simulink model "quadrotor"  (R2018b)
settings: Solver=ode4  StartTime=0.0  StopTime=inf  FixedStep=dt  RelTol=1e-3
values from neighbouring files (symbols this model uses):
  dt = 0.001    [InitSimulation.m]
  gravity = 9.81    [modelParameters.m]
  vehicle =     [Quadcopter-250mm-0.6kg-15min-EMAX.mat]    (also in Quadcopter-450mm-1.5kg-7min-DJI.mat)
libraries: simulink_extras x1

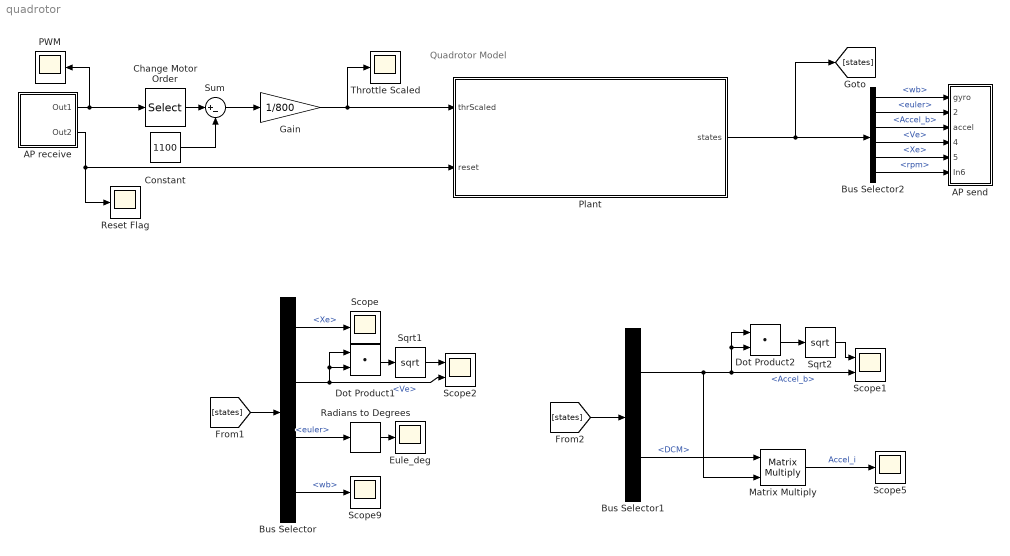
== system quadrotor ==
  note: Quadrotor Model
  AP receive : Subsystem  AncestorBlock=AP_Conector/AP receive
  AP send : Subsystem  AncestorBlock=AP_Conector/AP send
  Bus Selector : BusSelector  OutputSignals=Xe,Ve,euler,wb
  Bus Selector1 : BusSelector  OutputSignals=Accel_b,DCM
  Bus Selector2 : BusSelector  OutputSignals=wb,euler,Accel_b,Ve,Xe,rpm
  Change Motor Order : Selector  InputPortWidth=16  IndexOptions=Index vector (dialog)  Indices=[1 4 2 3]  OutputSizes=1
  Constant : Constant  Value=1100
  Dot Product1 : DotProduct  InputSameDT=on  OutDataTypeStr=Inherit: Inherit via internal rule
  Dot Product2 : DotProduct  InputSameDT=on  OutDataTypeStr=Inherit: Inherit via internal rule
  Eule_deg : Scope
  Gain : Gain  Gain=1/800
  Matrix Multiply : Product  Multiplication=Matrix(*)
  PWM : Scope
  Plant : Subsystem
  Radians to Degrees : simulink_extras/Transformations/Radians to Degrees
  Reset Flag : Scope
  Scope : Scope
  Scope1 : Scope  NumInputPorts=2
  Scope2 : Scope  NumInputPorts=2
  Scope5 : Scope
  Scope9 : Scope
  Sqrt1 : Sqrt  SaturateOnIntegerOverflow=on
  Sqrt2 : Sqrt  SaturateOnIntegerOverflow=on
  Sum : Sum  Inputs=|+-
  Throttle Scaled : Scope
  wires:
  [states] -> Bus Selector/1
  Bus Selector/1 -> Scope/1  "<Xe>"
  Bus Selector/2 -> Dot Product1/1, Dot Product1/2, Scope2/2  "<Ve>"
  Plant/1(states) -> [states], Bus Selector2/1
  Bus Selector/3 -> Radians to Degrees/1  "<euler>"
  Radians to Degrees/1 -> Eule_deg/1
  [states] -> Bus Selector1/1
  Bus Selector1/1 -> Scope1/2, Dot Product2/1, Dot Product2/2, Matrix Multiply/2  "<Accel_b>"
  Bus Selector/4 -> Scope9/1  "<wb>"
  Dot Product1/1 -> Sqrt1/1
  Sqrt1/1 -> Scope2/1
  Dot Product2/1 -> Sqrt2/1
  Sqrt2/1 -> Scope1/1
  AP receive/1(Out1) -> Change Motor Order/1, PWM/1
  Change Motor Order/1 -> Sum/1
  Bus Selector2/1 -> AP send/1(gyro)  "<wb>"
  Bus Selector2/2 -> AP send/2(attitude)  "<euler>"
  Bus Selector2/3 -> AP send/3(accel)  "<Accel_b>"
  Bus Selector2/4 -> AP send/4(velocity)  "<Ve>"
  Bus Selector2/5 -> AP send/5(position)  "<Xe>"
  Constant/1 -> Sum/2
  Sum/1 -> Gain/1
  Gain/1 -> Throttle Scaled/1, Plant/1(thrScaled)
  AP receive/2(Out2) -> Reset Flag/1, Plant/2(reset)
  Bus Selector1/2 -> Matrix Multiply/1  "<DCM>"
  Matrix Multiply/1 -> Scope5/1  "Accel_i"
  Bus Selector2/6 -> AP send/6(In6)  "<rpm>"

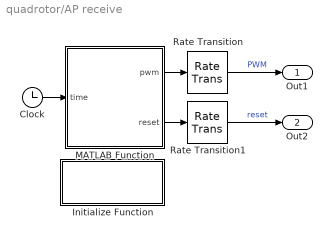
== system quadrotor/AP receive ==
  Clock : Clock
  Initialize Function : Subsystem  TreatAsAtomicUnit=on
  MATLAB Function : MATLAB Function  TreatAsAtomicUnit=on  SystemSampleTime=1/1000
  Rate Transition : RateTransition
  Rate Transition1 : RateTransition
  Out1 : Outport  VectorParamsAs1DForOutWhenUnconnected=on
  Out2 : Outport  Port=2  VectorParamsAs1DForOutWhenUnconnected=on
  wires:
  Rate Transition1/1 -> Out2/1  "reset"
  MATLAB Function/2(reset) -> Rate Transition1/1
  Clock/1 -> MATLAB Function/1(time)
  MATLAB Function/1(pwm) -> Rate Transition/1
  Rate Transition/1 -> Out1/1  "PWM"

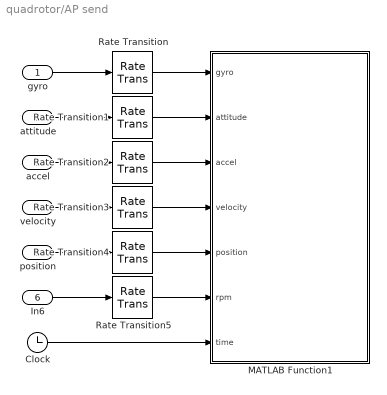
== system quadrotor/AP send ==
  gyro : Inport
  attitude : Inport  Port=2
  accel : Inport  Port=3
  velocity : Inport  Port=4
  position : Inport  Port=5
  In6 : Inport  Port=6
  Clock : Clock
  MATLAB Function1 : MATLAB Function  TreatAsAtomicUnit=on  SystemSampleTime=1/1000
  Rate Transition{,1..5} (6 alike) : RateTransition
  wires:
  position/1 -> Rate Transition4/1
  velocity/1 -> Rate Transition3/1
  Rate Transition4/1 -> MATLAB Function1/5(position)
  accel/1 -> Rate Transition2/1
  Rate Transition1/1 -> MATLAB Function1/2(attitude)
  Rate Transition2/1 -> MATLAB Function1/3(accel)
  Rate Transition3/1 -> MATLAB Function1/4(velocity)
  Clock/1 -> MATLAB Function1/7(time)
  Rate Transition/1 -> MATLAB Function1/1(gyro)
  gyro/1 -> Rate Transition/1
  attitude/1 -> Rate Transition1/1
  In6/1 -> Rate Transition5/1
  Rate Transition5/1 -> MATLAB Function1/6(rpm)

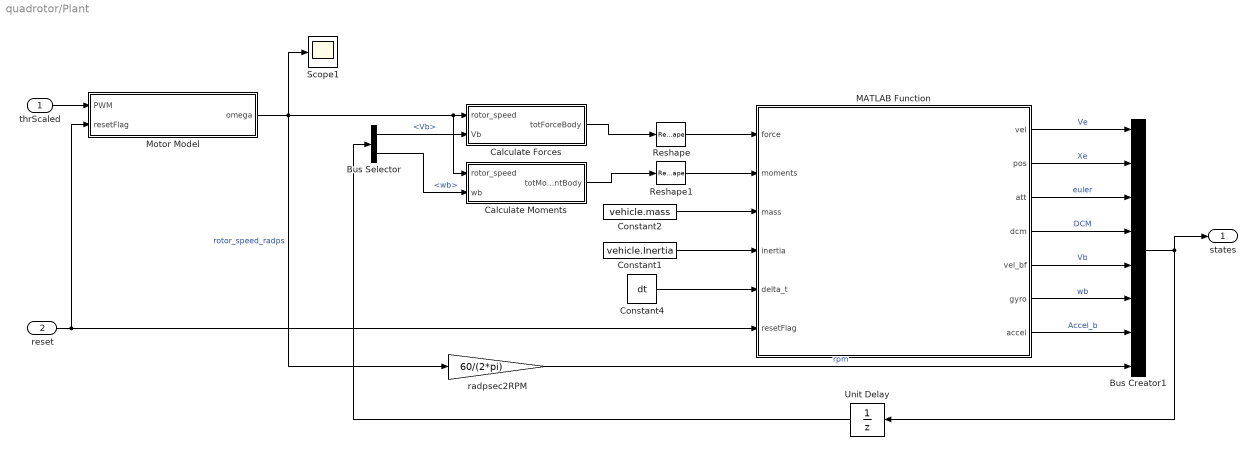
== system quadrotor/Plant ==
  thrScaled : Inport
  reset : Inport  Port=2
  Bus Creator1 : BusCreator  Inputs=8
  Bus Selector : BusSelector  OutputSignals=Vb,wb
  Calculate Forces : Subsystem
  Calculate Moments : Subsystem
  Constant1 : Constant  Value=vehicle.Inertia
  Constant2 : Constant  Value=vehicle.mass
  Constant4 : Constant  Value=dt
  MATLAB Function : MATLAB Function  TreatAsAtomicUnit=on
  Motor Model : Subsystem
  Reshape : Reshape  OutputDimensionality=Column vector (2-D)
  Reshape1 : Reshape  OutputDimensionality=Column vector (2-D)
  Scope1 : Scope
  Unit Delay : UnitDelay  SampleTime=-1
  radpsec2RPM : Gain  Gain=60/(2*pi)
  states : Outport
  wires:
  thrScaled/1 -> Motor Model/1(PWM)
  Motor Model/1(omega) -> Scope1/1, radpsec2RPM/1, Calculate Forces/1(rotor_speed), Calculate Moments/1(rotor_speed)  "rotor_speed_radps"
  Constant2/1 -> MATLAB Function/3(mass)
  Constant1/1 -> MATLAB Function/4(inertia)
  Constant4/1 -> MATLAB Function/5(delta_t)
  MATLAB Function/1(vel) -> Bus Creator1/1  "Ve"
  MATLAB Function/2(pos) -> Bus Creator1/2  "Xe"
  MATLAB Function/3(att) -> Bus Creator1/3  "euler"
  MATLAB Function/4(dcm) -> Bus Creator1/4  "DCM"
  MATLAB Function/5(vel_bf) -> Bus Creator1/5  "Vb"
  MATLAB Function/6(gyro) -> Bus Creator1/6  "wb"
  MATLAB Function/7(accel) -> Bus Creator1/7  "Accel_b"
  Bus Creator1/1 -> states/1, Unit Delay/1
  Reshape/1 -> MATLAB Function/1(force)
  Reshape1/1 -> MATLAB Function/2(moments)
  Calculate Forces/1(totForceBody) -> Reshape/1
  Calculate Moments/1(totMomentBody) -> Reshape1/1
  Unit Delay/1 -> Bus Selector/1
  radpsec2RPM/1 -> Bus Creator1/8  "rpm"
  Bus Selector/1 -> Calculate Forces/2(Vb)  "<Vb>"
  Bus Selector/2 -> Calculate Moments/2(wb)  "<wb>"
  reset/1 -> MATLAB Function/6(resetFlag), Motor Model/2(resetFlag)

== system quadrotor/AP receive/Initialize Function ==
  Event Listener : EventListener  DisableCoverage=on  EventName=reset
  Ground : Ground
  Ground1 : Ground
  Interpreted MATLAB Function : MATLABFcn  MATLABFcn=clear('AP_receive')  OutputDimensions=0
  Interpreted MATLAB Function1 : MATLABFcn  MATLABFcn=clear('AP_send')  OutputDimensions=0
  wires:
  Ground/1 -> Interpreted MATLAB Function/1
  Ground1/1 -> Interpreted MATLAB Function1/1

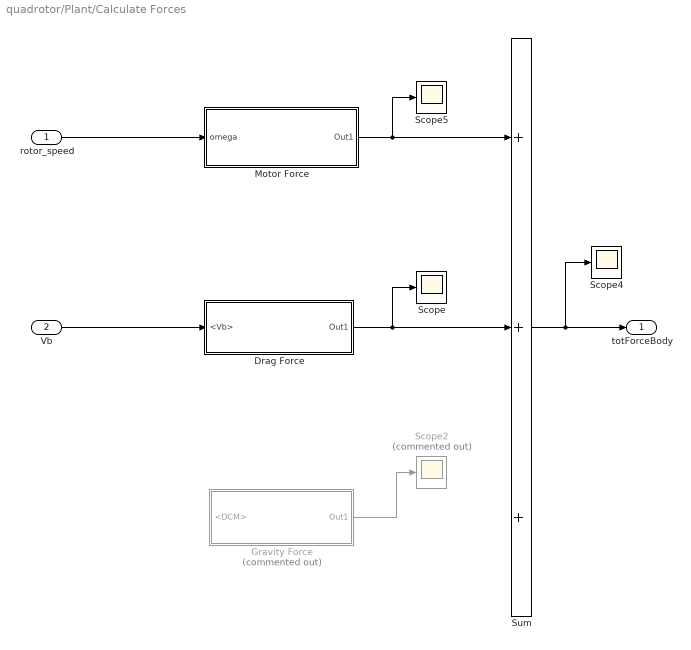
== system quadrotor/Plant/Calculate Forces ==
  rotor_speed : Inport
  Vb : Inport  Port=2
  Drag Force : Subsystem
  Gravity Force : Subsystem  Commented=on
  Motor Force : Subsystem
  Scope : Scope
  Scope2 : Scope  Commented=on
  Scope4 : Scope
  Scope5 : Scope
  Sum : Sum  Inputs=+++
  totForceBody : Outport
  wires:
  Sum/1 -> Scope4/1, totForceBody/1
  Vb/1 -> Drag Force/1(<Vb>)
  Drag Force/1(Out1) -> Sum/2, Scope/1
  Gravity Force/1(Out1) -> Scope2/1
  rotor_speed/1 -> Motor Force/1(omega)
  Motor Force/1(Out1) -> Scope5/1, Sum/1

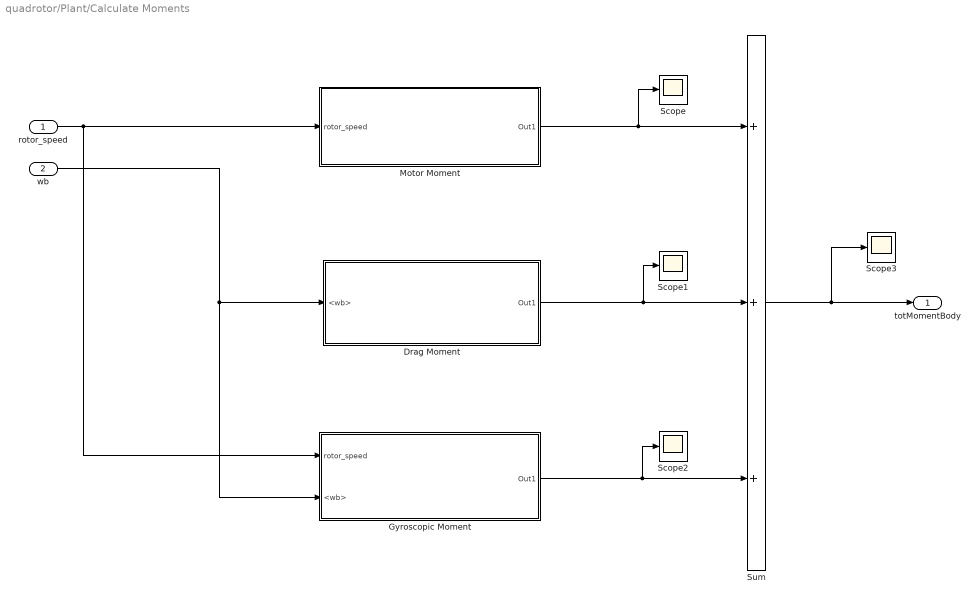
== system quadrotor/Plant/Calculate Moments ==
  rotor_speed : Inport
  wb : Inport  Port=2
  Drag Moment : Subsystem
  Gyroscopic Moment : Subsystem
  Motor Moment : Subsystem
  Scope{,1..3} (4 alike) : Scope
  Sum : Sum  Inputs=+++
  totMomentBody : Outport
  wires:
  rotor_speed/1 -> Gyroscopic Moment/1(rotor_speed), Motor Moment/1(rotor_speed)
  Sum/1 -> Scope3/1, totMomentBody/1
  Motor Moment/1(Out1) -> Scope/1, Sum/1
  Gyroscopic Moment/1(Out1) -> Sum/3, Scope2/1
  Drag Moment/1(Out1) -> Scope1/1, Sum/2
  wb/1 -> Gyroscopic Moment/2(<wb>), Drag Moment/1(<wb>)

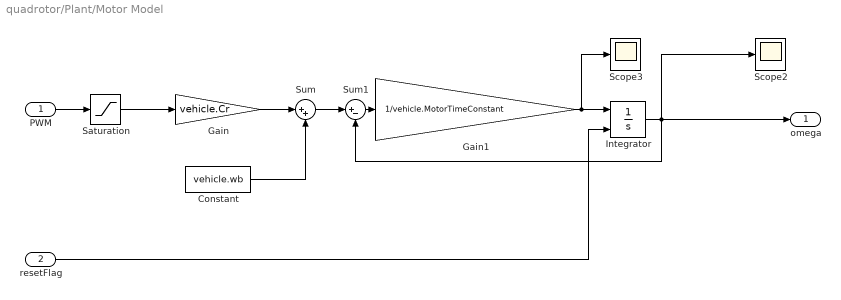
== system quadrotor/Plant/Motor Model ==
  PWM : Inport
  resetFlag : Inport  Port=2
  Constant : Constant  Value=vehicle.wb
  Gain : Gain  Gain=vehicle.Cr
  Gain1 : Gain  Gain=1/vehicle.MotorTimeConstant
  Integrator : Integrator  ExternalReset=rising  LimitOutput=on  UpperSaturationLimit=vehicle.Cr  LowerSaturationLimit=0
  Saturation : Saturate  UpperLimit=1  LowerLimit=0
  Scope2 : Scope
  Scope3 : Scope
  Sum : Sum  Inputs=|++
  Sum1 : Sum  Inputs=|+-
  omega : Outport
  wires:
  PWM/1 -> Saturation/1
  Saturation/1 -> Gain/1
  Gain/1 -> Sum/1
  Constant/1 -> Sum/2
  Sum/1 -> Sum1/1
  Sum1/1 -> Gain1/1
  Integrator/1 -> omega/1, Scope2/1, Sum1/2
  Gain1/1 -> Scope3/1, Integrator/1
  resetFlag/1 -> Integrator/2

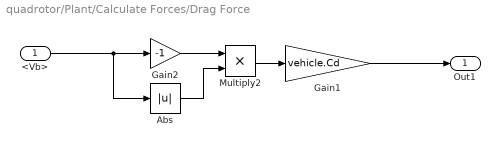
== system quadrotor/Plant/Calculate Forces/Drag Force ==
  <Vb> : Inport
  Abs : Abs
  Gain1 : Gain  Gain=vehicle.Cd
  Gain2 : Gain  Gain=-1
  Multiply2 : Product
  Out1 : Outport
  wires:
  <Vb>/1 -> Gain2/1, Abs/1
  Multiply2/1 -> Gain1/1
  Abs/1 -> Multiply2/2
  Gain2/1 -> Multiply2/1
  Gain1/1 -> Out1/1

== system quadrotor/Plant/Calculate Forces/Gravity Force ==
  <DCM> : Inport
  Constant1 : Constant  Value=[0; 0; gravity]
  Gain3 : Gain  Gain=vehicle.mass
  Matrix Multiply : Product  Multiplication=Matrix(*)
  Out1 : Outport
  wires:
  Constant1/1 -> Gain3/1
  Gain3/1 -> Matrix Multiply/2
  Matrix Multiply/1 -> Out1/1
  <DCM>/1 -> Matrix Multiply/1

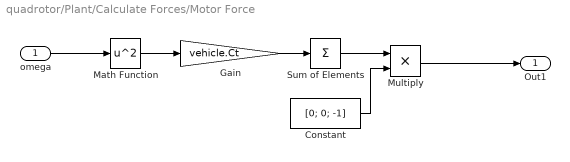
== system quadrotor/Plant/Calculate Forces/Motor Force ==
  omega : Inport
  Constant : Constant  Value=[0; 0; -1]
  Gain : Gain  Gain=vehicle.Ct
  Math Function : Math  Operator=square  SaturateOnIntegerOverflow=on
  Multiply : Product
  Sum of Elements : Sum  Inputs=+
  Out1 : Outport
  wires:
  omega/1 -> Math Function/1
  Sum of Elements/1 -> Multiply/1
  Multiply/1 -> Out1/1
  Constant/1 -> Multiply/2
  Math Function/1 -> Gain/1
  Gain/1 -> Sum of Elements/1

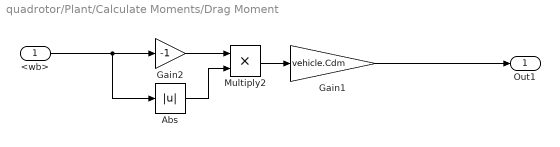
== system quadrotor/Plant/Calculate Moments/Drag Moment ==
  <wb> : Inport
  Abs : Abs
  Gain1 : Gain  Gain=vehicle.Cdm
  Gain2 : Gain  Gain=-1
  Multiply2 : Product
  Out1 : Outport
  wires:
  Abs/1 -> Multiply2/2
  Multiply2/1 -> Gain1/1
  <wb>/1 -> Abs/1, Gain2/1
  Gain2/1 -> Multiply2/1
  Gain1/1 -> Out1/1

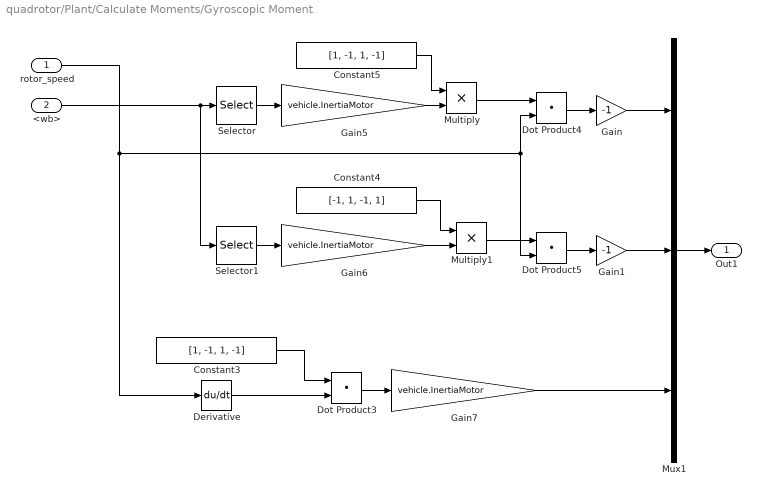
== system quadrotor/Plant/Calculate Moments/Gyroscopic Moment ==
  rotor_speed : Inport
  <wb> : Inport  Port=2
  Constant3 : Constant  Value=[1, -1, 1, -1]
  Constant4 : Constant  Value=[-1, 1, -1, 1]
  Constant5 : Constant  Value=[1, -1, 1, -1]
  Derivative : Derivative
  Dot Product3 : DotProduct  InputSameDT=on  OutDataTypeStr=Inherit: Inherit via internal rule
  Dot Product4 : DotProduct  InputSameDT=on  OutDataTypeStr=Inherit: Inherit via internal rule
  Dot Product5 : DotProduct  InputSameDT=on  OutDataTypeStr=Inherit: Inherit via internal rule
  Gain : Gain  Gain=-1
  Gain1 : Gain  Gain=-1
  Gain5 : Gain  Gain=vehicle.InertiaMotor
  Gain6 : Gain  Gain=vehicle.InertiaMotor
  Gain7 : Gain  Gain=vehicle.InertiaMotor
  Multiply : Product
  Multiply1 : Product
  Mux1 : Mux  Inputs=3
  Selector : Selector  InputPortWidth=3  IndexOptions=Index vector (dialog)  Indices=[2]  OutputSizes=1
  Selector1 : Selector  InputPortWidth=3  IndexOptions=Index vector (dialog)  Indices=[1]  OutputSizes=1
  Out1 : Outport
  wires:
  Selector1/1 -> Gain6/1
  Multiply1/1 -> Dot Product5/1
  Gain6/1 -> Multiply1/2
  Constant5/1 -> Multiply/1
  Dot Product4/1 -> Gain/1
  Constant3/1 -> Dot Product3/1
  Dot Product3/1 -> Gain7/1
  rotor_speed/1 -> Derivative/1, Dot Product5/2, Dot Product4/2
  Constant4/1 -> Multiply1/1
  Gain5/1 -> Multiply/2
  Selector/1 -> Gain5/1
  <wb>/1 -> Selector1/1, Selector/1
  Derivative/1 -> Dot Product3/2
  Multiply/1 -> Dot Product4/1
  Dot Product5/1 -> Gain1/1
  Mux1/1 -> Out1/1
  Gain/1 -> Mux1/1
  Gain1/1 -> Mux1/2
  Gain7/1 -> Mux1/3

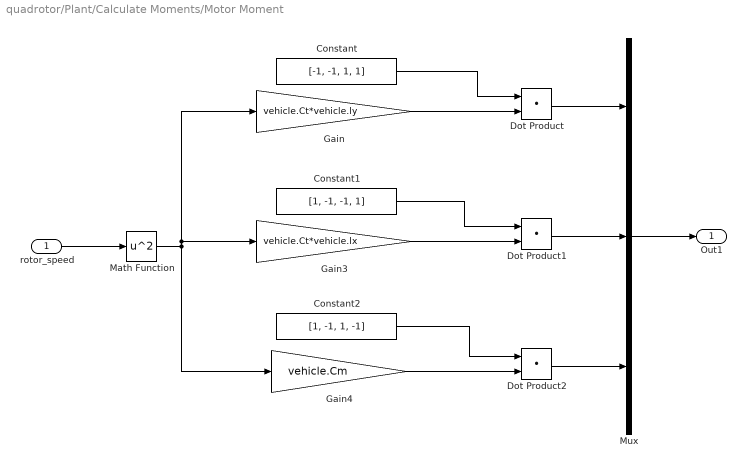
== system quadrotor/Plant/Calculate Moments/Motor Moment ==
  rotor_speed : Inport
  Constant : Constant  Value=[-1, -1, 1, 1]
  Constant1 : Constant  Value=[1, -1, -1, 1]
  Constant2 : Constant  Value=[1, -1, 1, -1]
  Dot Product : DotProduct  InputSameDT=on  OutDataTypeStr=Inherit: Inherit via internal rule
  Dot Product1 : DotProduct  InputSameDT=on  OutDataTypeStr=Inherit: Inherit via internal rule
  Dot Product2 : DotProduct  InputSameDT=on  OutDataTypeStr=Inherit: Inherit via internal rule
  Gain : Gain  Gain=vehicle.Ct*vehicle.ly
  Gain3 : Gain  Gain=vehicle.Ct*vehicle.lx
  Gain4 : Gain  Gain=vehicle.Cm
  Math Function : Math  Operator=square  SaturateOnIntegerOverflow=on
  Mux : Mux  Inputs=3
  Out1 : Outport
  wires:
  Gain/1 -> Dot Product/2
  Dot Product2/1 -> Mux/3
  Gain4/1 -> Dot Product2/2
  Math Function/1 -> Gain/1, Gain3/1, Gain4/1
  Gain3/1 -> Dot Product1/2
  Dot Product/1 -> Mux/1
  Constant2/1 -> Dot Product2/1
  Mux/1 -> Out1/1
  Constant/1 -> Dot Product/1
  Dot Product1/1 -> Mux/2
  Constant1/1 -> Dot Product1/1
  rotor_speed/1 -> Math Function/1

== matlab function quadrotor/AP receive/MATLAB Function ==
function [pwm, reset]  = fcn(time)
pwm = zeros(16,1); %#ok<PREALL>
reset = false; %#ok<NASGU>
coder.extrinsic('AP_receive')
[pwm, reset] = AP_receive(time);
end

== matlab function quadrotor/Plant/MATLAB Function ==
  settings: updateMethod=DISCRETE

% integrate the acceleration resulting from the forces and moments to get the
% new state
function [vel, pos, att, dcm, vel_bf, gyro, accel] = update_dynamics(force,moments, mass, inertia, delta_t, resetFlag)

persistent state
if isempty(state) || resetFlag
    state.gyro = [0;0;0]; % (rad/sec)
    state.dcm = diag([1,1,1]); % direction cosine matrix from body to inertial frame
    state.attitude = [0;0;0]; % (radians) (roll, pitch, yaw)
    state.accel = [0;0;0]; % (m/s^2) body frame
    state.velocity = [0;0;0]; % (m/s) earth frame
    state.position = [0;0;0]; % (m) earth frame
    state.bf_velo = [0;0;0]; % (m/s) body frame
    state.gravity_mss = 9.80665; % (m/s^2)
end

% inertia is inverted. check \ operator
rot_accel = inertia \ (moments - cross(state.gyro, inertia * state.gyro));
% rot_accel = ((moments)' / inertia)';

state.gyro = state.gyro + rot_accel * delta_t;

% Constrain to 2000 deg per second, this is what typical sensors max out at
state.gyro = max(state.gyro,deg2rad(-2000));
state.gyro = min(state.gyro,deg2rad(2000));

% update the dcm and attitude
[state.dcm, state.attitude] = rotate_dcm(state.dcm,state.gyro * delta_t);

% body frame accelerations
state.accel = force / mass;

% earth frame accelerations (NED)
accel_ef = state.dcm * state.accel;
accel_ef(3) = accel_ef(3) + state.gravity_mss;

% if we're on the ground, then our vertical acceleration is limited
% to zero. This effectively adds the force of the ground on the aircraft
if state.position(3) >= 0 && accel_ef(3) > 0
    accel_ef(3) = 0;
end

% work out acceleration as seen by the accelerometers. It sees the kinematic
% acceleration (ie. real movement), plus gravity
state.accel = state.dcm' * (accel_ef + [0; 0; -state.gravity_mss]);

state.velocity = state.velocity + accel_ef * delta_t;
state.position = state.position + state.velocity * delta_t;

% make sure we can't go underground (NED so underground is positive)
if state.position(3) >= 0
    state.position(3) = 0;
    state.velocity = [0;0;0];
    state.gyro = [0;0;0];
    state.attitude(1:2) = [0;0];
end

% calculate the body frame velocity for drag calculation
state.bf_velo = state.dcm' * state.velocity;

pos = state.position;
vel = state.velocity;
att = state.attitude;
gyro = state.gyro;
accel = state.accel;
vel_bf = state.bf_velo;
dcm = state.dcm;
end

function [dcm, euler] = rotate_dcm(dcm, ang)

% rotate
delta = [dcm(1,2) * ang(3) - dcm(1,3) * ang(2),         dcm(1,3) * ang(1) - dcm(1,1) * ang(3),      dcm(1,1) * ang(2) - dcm(1,2) * ang(1);
         dcm(2,2) * ang(3) - dcm(2,3) * ang(2),         dcm(2,3) * ang(1) - dcm(2,1) * ang(3),      dcm(2,1) * ang(2) - dcm(2,2) * ang(1);
         dcm(3,2) * ang(3) - dcm(3,3) * ang(2),         dcm(3,3) * ang(1) - dcm(3,1) * ang(3),      dcm(3,1) * ang(2) - dcm(3,2) * ang(1)];

dcm = dcm + delta;

% normalise
a = dcm(1,:);
b = dcm(2,:);
error = a * b';
t0 = a - (b *(0.5 * error));
t1 = b - (a *(0.5 * error));
t2 = cross(t0,t1);
dcm(1,:) = t0 * (1/norm(t0));
dcm(2,:) = t1 * (1/norm(t1));
dcm(3,:) = t2 * (1/norm(t2));

% calculate euler angles
euler = [atan2(dcm(3,2),dcm(3,3)); -asin(dcm(3,1)); atan2(dcm(2,1),dcm(1,1))]; 

end

== matlab function quadrotor/AP send/MATLAB Function1 ==
function fcn(gyro, attitude, accel, velocity, position, rpm, time)
coder.extrinsic('AP_send')
AP_send(gyro, attitude, accel, velocity, position, rpm, time)
end
